simulink model "roessler"  (Simulink 7.1)
settings: Solver=ode45  StartTime=0.0  StopTime=100  MaxStep=0.01  MinStep=0.001  RelTol=1e-3
libraries: simulink x1
settings Model: Creator=surbaniak  LastModifiedBy=surbaniak

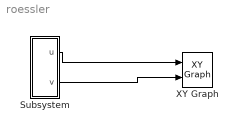
== system roessler ==
  Subsystem : Subsystem  mask{a=0.2, b=0.2, c=5.7}
  XY Graph : simulink/Sinks/XY Graph  SystemSampleTime=-1  xmin=-15  xmax=15  ymin=-10  ymax=25  st=-1
  wires:
  Subsystem/1(u) -> XY Graph/1
  Subsystem/2(v) -> XY Graph/2

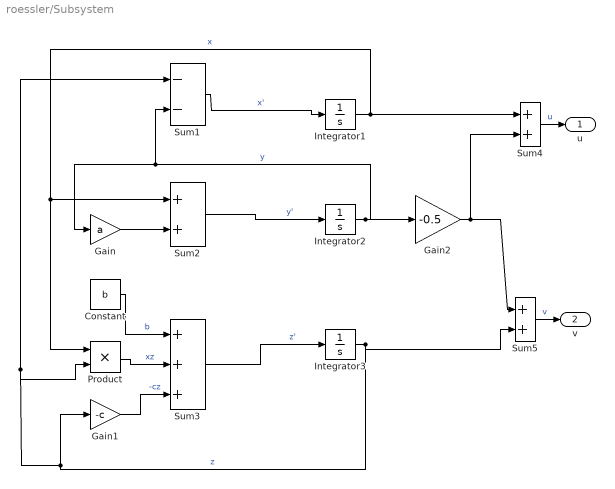
== system roessler/Subsystem ==
  Constant : Constant  Value=b  OutDataType=sfix(16)  OutScaling=2^0
  Gain : Gain  Gain=a  ParameterDataType=sfix(16)  ParameterScaling=2^0  OutDataType=sfix(16)  OutScaling=2^0
  Gain1 : Gain  Gain=-c  ParameterDataType=sfix(16)  ParameterScaling=2^0  OutDataType=sfix(16)  OutScaling=2^0
  Gain2 : Gain  Gain=-0.5  ParameterDataType=sfix(16)  ParameterScaling=2^0  OutDataType=sfix(16)  OutScaling=2^0
  Integrator1 : Integrator
  Integrator2 : Integrator
  Integrator3 : Integrator
  Product : Product  OutDataType=sfix(16)  OutScaling=2^0  RndMeth=Zero
  Sum1 : Sum  Inputs=--  OutDataType=sfix(16)  OutScaling=2^0
  Sum2 : Sum  OutDataType=sfix(16)  OutScaling=2^0
  Sum3 : Sum  Inputs=+++  OutDataType=sfix(16)  OutScaling=2^0
  Sum4 : Sum  OutDataType=sfix(16)  OutScaling=2^0
  Sum5 : Sum  OutDataType=sfix(16)  OutScaling=2^0
  u : Outport
  v : Outport  Port=2
  wires:
  Integrator2/1 -> Sum1/2, Gain/1, Gain2/1  "y"
  Integrator3/1 -> Gain1/1, Sum1/1, Product/2, Sum5/2  "z"
  Sum1/1 -> Integrator1/1  "x'"
  Gain/1 -> Sum2/2
  Integrator1/1 -> Sum2/1, Product/1, Sum4/1  "x"
  Sum2/1 -> Integrator2/1  "y'"
  Sum3/1 -> Integrator3/1  "z'"
  Gain1/1 -> Sum3/3  "-cz"
  Constant/1 -> Sum3/1  "b"
  Product/1 -> Sum3/2  "xz"
  Gain2/1 -> Sum4/2, Sum5/1
  Sum4/1 -> u/1  "u"
  Sum5/1 -> v/1  "v"
